simulink model "DC_7b"  (R2022b)
settings: Solver=VariableStepAuto  StartTime=0.0  StopTime=t_sim  RelTol=1e-3
undefined symbols (not defined in the file or in its folder): d1, ts
libraries: cstblocks x3, simulink x1
settings Model: Creator=alici  LastModifiedBy=alici

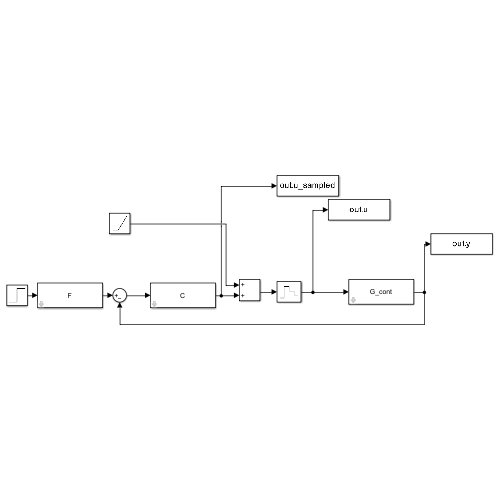
[thumbnail: Simulink's stored preview of the top-level diagram]
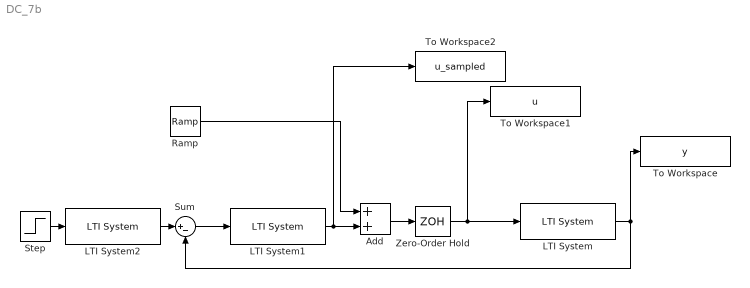
== system DC_7b ==
  Add : Sum
  LTI System : cstblocks/LTI System  sys=G_cont  IC=[]
  LTI System1 : cstblocks/LTI System  sys=C  IC=[]
  LTI System2 : cstblocks/LTI System  sys=F  IC=[]
  Ramp : simulink/Sources/Ramp  slope=d1  start=0  InitialOutput=0
  Step : Step  Time=0  SampleTime=0
  Sum : Sum  Inputs=|+-
  To Workspace : ToWorkspace  VariableName=y  SaveFormat=Timeseries  SampleTime=ts/1000
  To Workspace1 : ToWorkspace  VariableName=u  SaveFormat=Timeseries  SampleTime=ts/1000
  To Workspace2 : ToWorkspace  VariableName=u_sampled  SaveFormat=Timeseries  SampleTime=ts
  Zero-Order Hold : ZeroOrderHold  SampleTime=ts
  wires:
  Sum/1 -> LTI System1/1
  LTI System/1 -> Sum/2, To Workspace/1
  LTI System2/1 -> Sum/1
  Step/1 -> LTI System2/1
  Ramp/1 -> Add/1
  LTI System1/1 -> To Workspace2/1, Add/2
  Add/1 -> Zero-Order Hold/1
  Zero-Order Hold/1 -> To Workspace1/1, LTI System/1
